simulink model "Lab3_Simulation"  (R2016a)
settings: Solver=VariableStepAuto  StartTime=0.0  StopTime=2  MaxStep=0.001  RelTol=1e-3
settings Model: Creator=Tomas  LastModifiedBy=Tomas

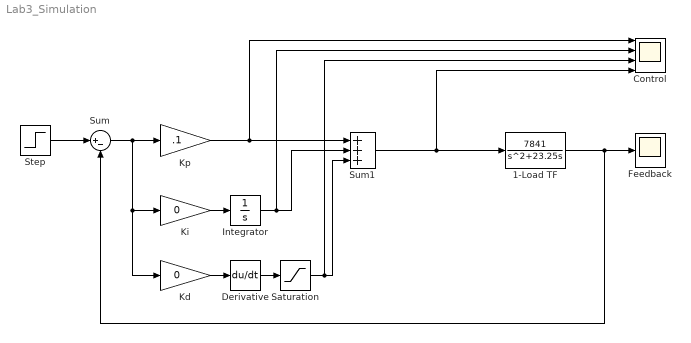
== system Lab3_Simulation ==
  1-Load TF : TransferFcn  Numerator=[7841]  Denominator=[1 23.25 0]
  Control : Scope  NumInputPorts=4
  Derivative : Derivative
  Feedback : Scope
  Integrator : Integrator
  Kd : Gain  Gain=0
  Ki : Gain  Gain=0
  Kp : Gain  Gain=.1
  Saturation : Saturate  UpperLimit=12  LowerLimit=-12
  Step : Step  After=45  SampleTime=0
  Sum : Sum  Inputs=|+-
  Sum1 : Sum  Inputs=+++
  wires:
  Step/1 -> Sum/1
  Sum/1 -> Kd/1, Ki/1, Kp/1
  Ki/1 -> Integrator/1
  Kp/1 -> Control/1, Sum1/1
  Integrator/1 -> Control/2, Sum1/2
  1-Load TF/1 -> Feedback/1, Sum/2
  Kd/1 -> Derivative/1
  Derivative/1 -> Saturation/1
  Sum1/1 -> Control/4, 1-Load TF/1
  Saturation/1 -> Control/3, Sum1/3
